simulink model "segmentImage"  (R2021a)
settings: Solver=VariableStepAuto  StartTime=0.0  StopTime=10  RelTol=1e-3
libraries: visionsources x1
settings Model: Creator=lipingw  LastModifiedBy=mmordeka
settings SolverCC: AlgebraicLoopSolver=TrustRegion
settings DebuggingCC: SFMachineParentedDataDiag=warning

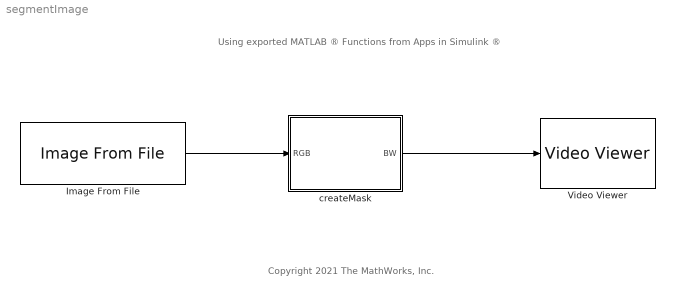
== system segmentImage ==
  note: Using exported MATLAB ® Functions from Apps
      | in Simulink ®
  note: Copyright 2021 The MathWorks, Inc.
  Image From File : visionsources/Image From File  Tag=vipblks_nd  FileName=frontViewRgbCrop.jpg  Ts=inf  imagePorts=One multidimensional signal  OutPortLabels=R|G|B  ImageDataType=Inherit from input image  sdImageDataType=uint(8)  Signed=on  WordLength=16  FractionLengthMode=User-defined  FractionLength=15
  Video Viewer : VideoViewer  FigPos=[1842 1269 1311 743]
  createMask : MATLAB Function  TreatAsAtomicUnit=on
  wires:
  Image From File/1 -> createMask/1(RGB)
  createMask/1(BW) -> Video Viewer/1

== matlab function segmentImage/createMask ==
  data: RGB input; BW output
function BW  = createMask(RGB)
%createMask  Threshold RGB image using auto-generated code from colorThresholder app.
%  [BW,MASKEDRGBIMAGE] = createMask(RGB) thresholds image RGB using
%  auto-generated code from the colorThresholder app. The colorspace and
%  range for each channel of the colorspace were set within the app. The
%  segmentation mask is returned in BW, and a composite of the mask and
%  original RGB images is returned in maskedRGBImage.

% Auto-generated by colorThresholder app on 11-Nov-2020
%------------------------------------------------------


% Convert RGB image to chosen color space
I = RGB;

% Define thresholds for channel 1 based on histogram settings
channel1Min = 222.000;
channel1Max = 255.000;

% Define thresholds for channel 2 based on histogram settings
channel2Min = 0.000;
channel2Max = 255.000;

% Define thresholds for channel 3 based on histogram settings
channel3Min = 0.000;
channel3Max = 145.000;

% Create mask based on chosen histogram thresholds
sliderBW = (I(:,:,1) >= channel1Min ) & (I(:,:,1) <= channel1Max) & ...
    (I(:,:,2) >= channel2Min ) & (I(:,:,2) <= channel2Max) & ...
    (I(:,:,3) >= channel3Min ) & (I(:,:,3) <= channel3Max);
BW = sliderBW;

end
